simulink model "crazyflie"  (R2021b)
settings: Solver=FixedStepDiscrete  StartTime=0.0  StopTime=160  FixedStep=0.001  RelTol=1e-3
undefined symbols (not defined in the file): DiscIntNeverNeededParam
settings Model: PauseTimes=7  Creator=Zrean  LastModifiedBy=bober2
settings SolverCC: AlgebraicLoopSolver=TrustRegion
settings DataIOCC: ReturnWorkspaceOutputs=off
settings OptimizationCC: DefaultParameterBehavior=Inlined  UseDivisionForNetSlopeComputation=on  UseFloatMulNetSlope=on  UseSpecifiedMinMax=on  InlineInvariantSignals=on  PassReuseOutputArgsAs=Individual arguments  ZeroExternalMemoryAtStartup=off  ZeroInternalMemoryAtStartup=off  NoFixptDivByZeroProtection=on  EfficientFloat2IntCast=on  LifeSpan=1  EfficientTunableParamExpr=on
settings DebuggingCC: AlgebraicLoopMsg=error  ParameterTunabilityLossMsg=error  ArithmeticOperatorsInVariantConditions=warning
settings HardwareCC: ProdBitPerPointer=32  ProdBitPerSizeT=32  ProdBitPerPtrDiffT=32  ProdLargestAtomicInteger=Long  ProdLargestAtomicFloat=Double  ProdWordSize=32  ProdHWDeviceType=ARM Compatible->ARM Cortex
settings SFSimCC: SimUseLocalCustomCode=off  MATLABDynamicMemAlloc=off  CustomCodeUndefinedFunction=UseInterfaceOnly
settings RTWCC: Description=Embedded Coder  SystemTargetFile=ert.tlc  GenCodeOnly=on  TemplateMakefile=ert_default_tmf  GenerateReport=on  RTWUseLocalCustomCode=off  BuildConfiguration=Faster Runs  IncludeHyperlinkInReport=on  LaunchReport=on  GenerateTraceInfo=on  GenerateTraceReport=on  GenerateTraceReportSl=on  GenerateTraceReportSf=on  GenerateTraceReportEml=on  GenerateCodeMetricsReport=on  DLArmComputeVersion=20.02.1
settings CodeAppCC: ForceParamTrailComments=on  IgnoreCustomStorageClasses=off  OperatorAnnotations=on  SimulinkDataObjDesc=on  SFDataObjDesc=on  MATLABFcnDesc=on  InsertBlockDesc=on  StateflowObjectComments=on  MATLABSourceComments=on
settings ERTTargetCC: TargetLangStandard=C99 (ISO)  MultiwordLength=2048  CombineSignalStateStructs=on  SuppressErrorStatus=on  SupportAbsoluteTime=off  SupportNonFinite=off  SupportComplex=off  InlinedParameterPlacement=NonHierarchical  ERTCustomFileTemplate=crazyflie_wrapper.tlc  ERTFilePackagingFormat=CompactWithDataFile
settings SimscapeCC: SimscapeNormalizeSystem=off

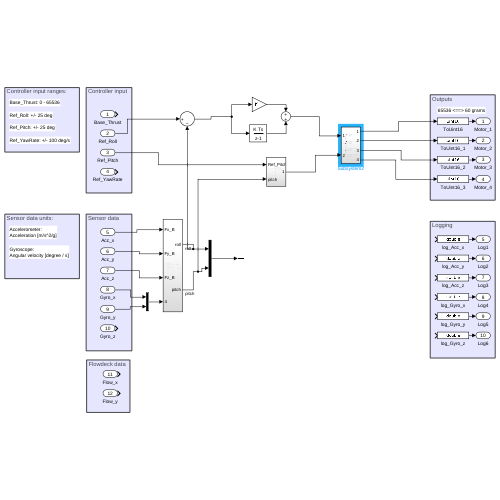
[thumbnail: Simulink's stored preview of the top-level diagram]
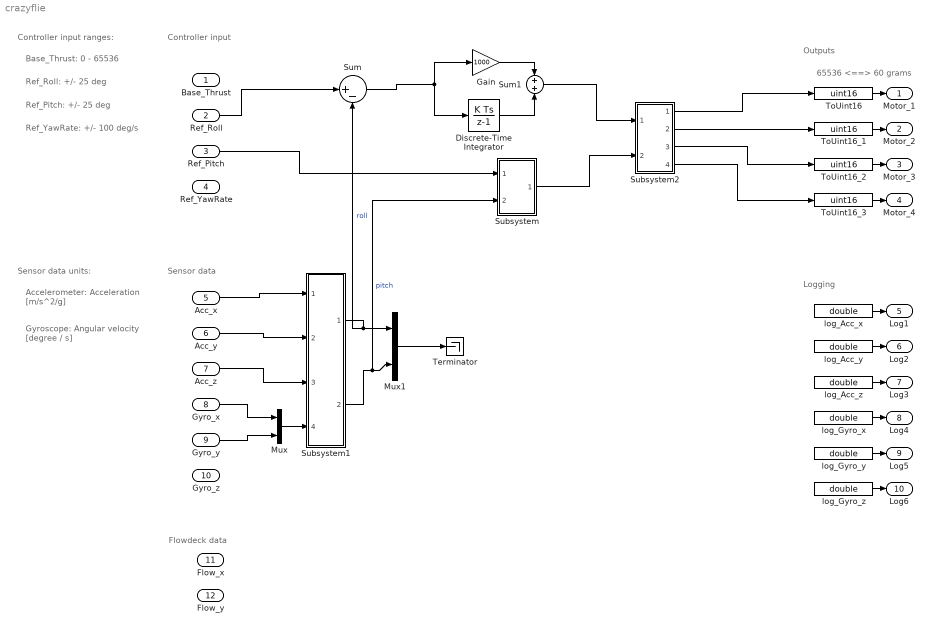
== system crazyflie ==
  note: 65536 <==> 60 grams
  note: Logging
  note: Outputs
  note: Sensor data
  note: Controller input
  note: Ref_Roll: +/- 25 deg
  note: Base_Thrust: 0 - 65536
  note: Ref_Pitch: +/- 25 deg
  note: Ref_YawRate: +/- 100 deg/s
  note: Controller input ranges:
  note: Gyroscope:
      | Angular velocity [degree / s]
  note: Accelerometer:
      | Acceleration [m/s^2/g]
  note: Sensor data units:
  note: Flowdeck data
  Base_Thrust : Inport  OutDataTypeStr=double
  Ref_Roll : Inport  Port=2  OutDataTypeStr=double
  Ref_Pitch : Inport  Port=3  OutDataTypeStr=double
  Ref_YawRate : Inport  Port=4  OutDataTypeStr=double
  Acc_x : Inport  Port=5  OutDataTypeStr=double  PortDimensions=1
  Acc_y : Inport  Port=6  OutDataTypeStr=double  PortDimensions=1
  Acc_z : Inport  Port=7  OutDataTypeStr=double  PortDimensions=1
  Gyro_x : Inport  Port=8  OutDataTypeStr=double  PortDimensions=1
  Gyro_y : Inport  Port=9  OutDataTypeStr=double  PortDimensions=1
  Gyro_z : Inport  Port=10  OutDataTypeStr=double  PortDimensions=1
  Flow_x : Inport  Port=11  OutDataTypeStr=int16  PortDimensions=1
  Flow_y : Inport  Port=12  OutDataTypeStr=int16  PortDimensions=1
  Discrete-Time Integrator : DiscreteIntegrator  SampleTime=-1  ICPrevOutput=DiscIntNeverNeededParam  ICPrevScaledInput=DiscIntNeverNeededParam
  Gain : Gain  Gain=1000
  Mux : Mux  Inputs=2
  Mux1 : Mux  Inputs=2
  Subsystem : Subsystem
  Subsystem1 : Subsystem
  Subsystem2 : Subsystem
  Sum : Sum  Inputs=|+-
  Sum1 : Sum
  Terminator : Terminator
  ToUint16 : DataTypeConversion  OutDataTypeStr=uint16  SaturateOnIntegerOverflow=on
  ToUint16_1 : DataTypeConversion  OutDataTypeStr=uint16  SaturateOnIntegerOverflow=on
  ToUint16_2 : DataTypeConversion  OutDataTypeStr=uint16  SaturateOnIntegerOverflow=on
  ToUint16_3 : DataTypeConversion  OutDataTypeStr=uint16  SaturateOnIntegerOverflow=on
  log_Acc_x : DataTypeConversion  OutDataTypeStr=double  SaturateOnIntegerOverflow=on
  log_Acc_y : DataTypeConversion  OutDataTypeStr=double  SaturateOnIntegerOverflow=on
  log_Acc_z : DataTypeConversion  OutDataTypeStr=double  SaturateOnIntegerOverflow=on
  log_Gyro_x : DataTypeConversion  OutDataTypeStr=double  SaturateOnIntegerOverflow=on
  log_Gyro_y : DataTypeConversion  OutDataTypeStr=double  SaturateOnIntegerOverflow=on
  log_Gyro_z : DataTypeConversion  OutDataTypeStr=double  SaturateOnIntegerOverflow=on
  Motor_1 : Outport  OutDataTypeStr=uint16  VectorParamsAs1DForOutWhenUnconnected=off  LockScale=on
  Motor_2 : Outport  Port=2  OutDataTypeStr=uint16  VectorParamsAs1DForOutWhenUnconnected=off  LockScale=on
  Motor_3 : Outport  Port=3  OutDataTypeStr=uint16  VectorParamsAs1DForOutWhenUnconnected=off  LockScale=on
  Motor_4 : Outport  Port=4  OutDataTypeStr=uint16  VectorParamsAs1DForOutWhenUnconnected=off  LockScale=on
  Log1 : Outport  Port=5  OutDataTypeStr=double  VectorParamsAs1DForOutWhenUnconnected=off
  Log2 : Outport  Port=6  OutDataTypeStr=double  VectorParamsAs1DForOutWhenUnconnected=off
  Log3 : Outport  Port=7  OutDataTypeStr=double  VectorParamsAs1DForOutWhenUnconnected=off
  Log4 : Outport  Port=8  OutDataTypeStr=double  VectorParamsAs1DForOutWhenUnconnected=off
  Log5 : Outport  Port=9  OutDataTypeStr=double  VectorParamsAs1DForOutWhenUnconnected=off
  Log6 : Outport  Port=10  OutDataTypeStr=double  VectorParamsAs1DForOutWhenUnconnected=off
  wires:
  ToUint16/1 -> Motor_1/1
  ToUint16_1/1 -> Motor_2/1
  ToUint16_2/1 -> Motor_3/1
  ToUint16_3/1 -> Motor_4/1
  log_Acc_x/1 -> Log1/1
  log_Acc_y/1 -> Log2/1
  log_Acc_z/1 -> Log3/1
  log_Gyro_x/1 -> Log4/1
  log_Gyro_y/1 -> Log5/1
  log_Gyro_z/1 -> Log6/1
  Gyro_x/1 -> Mux/1
  Gyro_y/1 -> Mux/2
  Acc_x/1 -> Subsystem1/1(Fx_B)
  Acc_y/1 -> Subsystem1/2(Fy_B)
  Acc_z/1 -> Subsystem1/3(Fz_B)
  Mux/1 -> Subsystem1/4(In4)
  Subsystem1/2(pitch) -> Subsystem/2(pitch), Mux1/2  "pitch"
  Ref_Roll/1 -> Sum/1
  Sum/1 -> Discrete-Time Integrator/1, Gain/1
  Gain/1 -> Sum1/1
  Discrete-Time Integrator/1 -> Sum1/2
  Subsystem1/1(roll) -> Mux1/1, Sum/2  "roll"
  Ref_Pitch/1 -> Subsystem/1(Ref_Pitch)
  Mux1/1 -> Terminator/1
  Sum1/1 -> Subsystem2/1(In1)
  Subsystem/1(Out1) -> Subsystem2/2(In2)
  Subsystem2/1(Out1) -> ToUint16/1
  Subsystem2/2(Out2) -> ToUint16_1/1
  Subsystem2/3(Out3) -> ToUint16_2/1
  Subsystem2/4(Out4) -> ToUint16_3/1

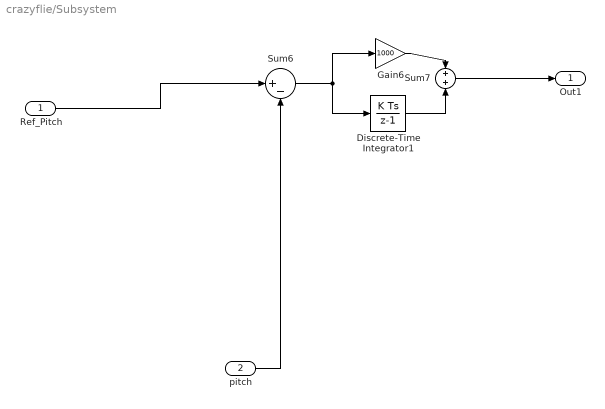
== system crazyflie/Subsystem ==
  Ref_Pitch : Inport
  pitch : Inport  Port=2
  Discrete-Time Integrator1 : DiscreteIntegrator  SampleTime=-1  ICPrevOutput=DiscIntNeverNeededParam  ICPrevScaledInput=DiscIntNeverNeededParam
  Gain6 : Gain  Gain=1000
  Sum6 : Sum  Inputs=|+-
  Sum7 : Sum
  Out1 : Outport
  wires:
  Ref_Pitch/1 -> Sum6/1
  Gain6/1 -> Sum7/1
  Discrete-Time Integrator1/1 -> Sum7/2
  Sum7/1 -> Out1/1
  pitch/1 -> Sum6/2
  Sum6/1 -> Discrete-Time Integrator1/1, Gain6/1

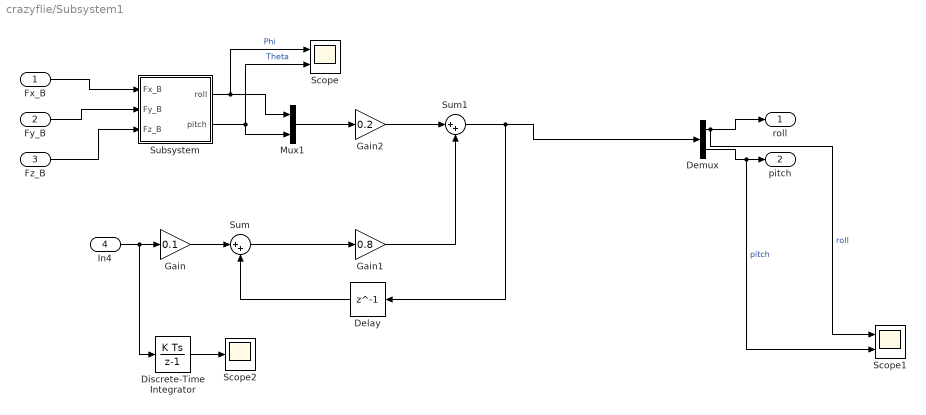
== system crazyflie/Subsystem1 ==
  Fx_B : Inport
  Fy_B : Inport  Port=2
  Fz_B : Inport  Port=3
  In4 : Inport  Port=4
  Delay : Delay  DelayLength=1
  Demux : Demux  Outputs=2
  Discrete-Time Integrator : DiscreteIntegrator  SampleTime=-1  ICPrevOutput=DiscIntNeverNeededParam  ICPrevScaledInput=DiscIntNeverNeededParam
  Gain : Gain  Gain=0.1
  Gain1 : Gain  Gain=0.8
  Gain2 : Gain  Gain=0.2
  Mux1 : Mux  Inputs=2
  Scope : Scope  NumInputPorts=2
  Scope1 : Scope  NumInputPorts=2
  Scope2 : Scope
  Subsystem : Subsystem
  Sum : Sum  Inputs=|++
  Sum1 : Sum  Inputs=|++
  roll : Outport
  pitch : Outport  Port=2
  wires:
  In4/1 -> Discrete-Time Integrator/1, Gain/1
  Mux1/1 -> Gain2/1
  Subsystem/1(roll) -> Scope/1, Mux1/1  "Phi"
  Subsystem/2(pitch) -> Scope/2, Mux1/2  "Theta"
  Fx_B/1 -> Subsystem/1(Fx_B)
  Fy_B/1 -> Subsystem/2(Fy_B)
  Fz_B/1 -> Subsystem/3(Fz_B)
  Sum1/1 -> Delay/1, Demux/1
  Gain2/1 -> Sum1/1
  Gain1/1 -> Sum1/2
  Gain/1 -> Sum/1
  Sum/1 -> Gain1/1
  Delay/1 -> Sum/2
  Demux/2 -> Scope1/2, pitch/1  "pitch"
  Demux/1 -> Scope1/1, roll/1  "roll"
  Discrete-Time Integrator/1 -> Scope2/1

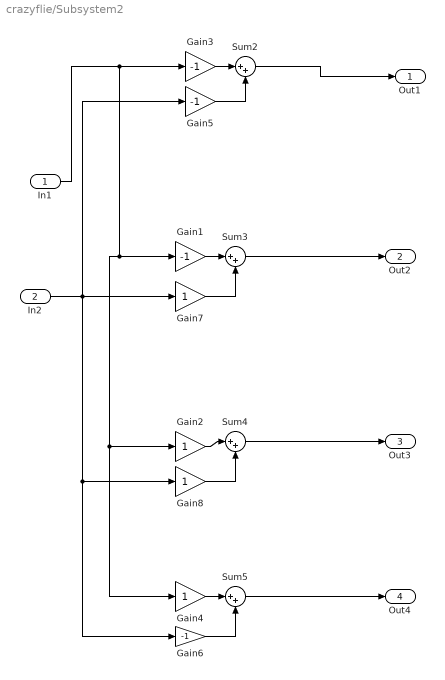
== system crazyflie/Subsystem2 ==
  In1 : Inport
  In2 : Inport  Port=2
  Gain{1,3,5..6} (4 alike) : Gain  Gain=-1
  Gain{2,4,7..8} (4 alike) : Gain
  Sum{2..5} (4 alike) : Sum  Inputs=|++
  Out1 : Outport
  Out2 : Outport  Port=2
  Out3 : Outport  Port=3
  Out4 : Outport  Port=4
  wires:
  Gain7/1 -> Sum3/2
  Gain4/1 -> Sum5/1
  Gain3/1 -> Sum2/1
  Sum2/1 -> Out1/1
  In1/1 -> Gain4/1, Gain2/1, Gain1/1, Gain3/1
  Gain8/1 -> Sum4/2
  Sum5/1 -> Out4/1
  Gain2/1 -> Sum4/1
  Gain1/1 -> Sum3/1
  In2/1 -> Gain6/1, Gain8/1, Gain7/1, Gain5/1
  Gain5/1 -> Sum2/2
  Gain6/1 -> Sum5/2
  Sum4/1 -> Out3/1
  Sum3/1 -> Out2/1

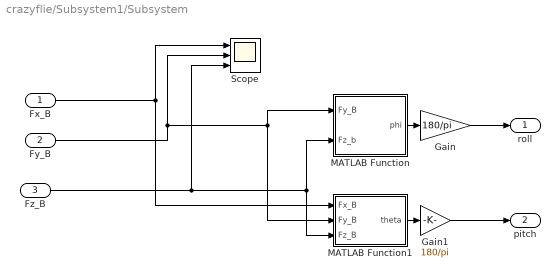
== system crazyflie/Subsystem1/Subsystem ==
  Fx_B : Inport
  Fy_B : Inport  Port=2
  Fz_B : Inport  Port=3
  Gain : Gain  Gain=180/pi
  Gain1 : Gain  Gain=180/pi
  MATLAB Function : MATLAB Function  TreatAsAtomicUnit=on
  MATLAB Function1 : MATLAB Function  TreatAsAtomicUnit=on
  Scope : Scope  NumInputPorts=3
  roll : Outport
  pitch : Outport  Port=2
  wires:
  MATLAB Function/1(phi) -> Gain/1
  MATLAB Function1/1(theta) -> Gain1/1
  Gain/1 -> roll/1
  Gain1/1 -> pitch/1
  Fx_B/1 -> Scope/1, MATLAB Function1/1(Fx_B)
  Fy_B/1 -> Scope/2, MATLAB Function/1(Fy_B), MATLAB Function1/2(Fy_B)
  Fz_B/1 -> Scope/3, MATLAB Function/2(Fz_b), MATLAB Function1/3(Fz_B)

== matlab function crazyflie/Subsystem1/Subsystem/MATLAB Function ==
  data: Fy_B input; phi output; Fz_b input
function phi = fcn(Fy_B,Fz_b)

phi= atan2(Fy_B,Fz_b);

== matlab function crazyflie/Subsystem1/Subsystem/MATLAB Function1 ==
  data: Fx_B input; Fy_B input; theta output; Fz_B input
function theta = fcn(Fx_B,Fy_B,Fz_B)
% fx or -fx ????
theta = atan2(-Fx_B,sqrt((Fy_B)^2+(Fz_B)^2));
